simulink model "OptiTrack_Example"  (R2023b)
settings: Solver=FixedStepAuto  StartTime=0.0  StopTime=inf  FixedStep=1/240  RelTol=1e-3
libraries: sharedtransform x1
settings Model: Creator=Rafael  LastModifiedBy=Rafael
settings OptimizationCC: ZeroExternalMemoryAtStartup=off  ZeroInternalMemoryAtStartup=off
settings RTWCC: TargetLang=C++
settings GRTTargetCC: TargetLangStandard=C++11 (ISO)  CodeInterfacePackaging=C++ class

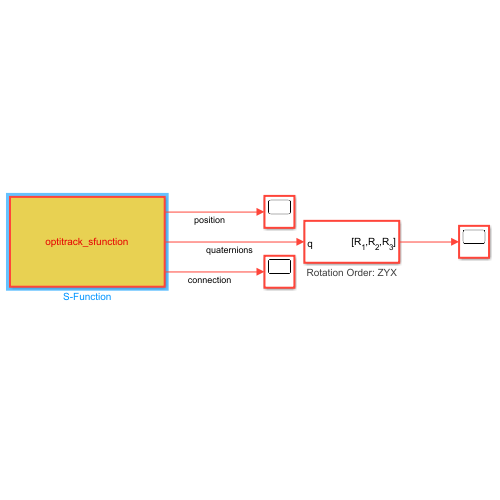
[thumbnail: Simulink's stored preview of the top-level diagram]
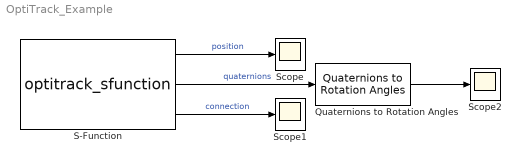
== system OptiTrack_Example ==
  Quaternions to Rotation Angles : sharedtransform/Quaternions to Rotation Angles  rotationOrder=ZYX  aMode=aMode
  S-Function : S-Function  FunctionName=optitrack_sfunction  Parameters='158.42.170.216', '158.42.46.62', 19  SFunctionDeploymentMode=off  EnableBusSupport=off
  Scope : Scope
  Scope1 : Scope
  Scope2 : Scope
  wires:
  S-Function/1 -> Scope/1  "position"
  S-Function/2 -> Quaternions to Rotation Angles/1  "quaternions"
  S-Function/3 -> Scope1/1  "connection"
  Quaternions to Rotation Angles/1 -> Scope2/1
